simulink model "o1_ar_filter"  (R2020b)
settings: Solver=FixedStepDiscrete  StartTime=0.0  StopTime=stopTime  RelTol=1e-3
undefined symbols (not defined in the file or in its folder): fs
settings Model: Creator=Ross  LastModifiedBy=conno
settings DataIOCC: SaveOutput=off  SaveTime=off  ReturnWorkspaceOutputs=off
settings OptimizationCC: BlockReduction=off  ConditionallyExecuteInputs=off  DefaultParameterBehavior=Inlined
settings DebuggingCC: ReadBeforeWriteMsg=DisableAll  WriteAfterWriteMsg=DisableAll  WriteAfterReadMsg=DisableAll  AlgebraicLoopMsg=error  MultiTaskDSMMsg=none  SingleTaskRateTransMsg=error  PregeneratedLibrarySubsystemCodeDiagnostic=none  ArithmeticOperatorsInVariantConditions=warning
settings HardwareCC: ProdBitPerPointer=32  ProdBitPerSizeT=32  ProdBitPerPtrDiffT=32  ProdLargestAtomicFloat=None  ProdIntDivRoundTo=Undefined  ProdEndianess=Unspecified  ProdWordSize=32  ProdHWDeviceType=ASIC/FPGA->ASIC/FPGA  TargetBitPerPointer=64  TargetBitPerSizeT=64  TargetBitPerPtrDiffT=64  TargetLongLongMode=on  TargetIntDivRoundTo=Zero  TargetEndianess=LittleEndian  TargetWordSize=64  TargetHWDeviceType=Custom Processor->MATLAB Host Computer  ProdEqTarget=off
settings ModelReferenceCC: UpdateModelReferenceTargets=IfOutOfDate
settings SFSimCC: SFSimEcho=off  SimUseLocalCustomCode=off  CustomCodeUndefinedFunction=UseInterfaceOnly
settings RTWCC: RTWUseLocalCustomCode=off

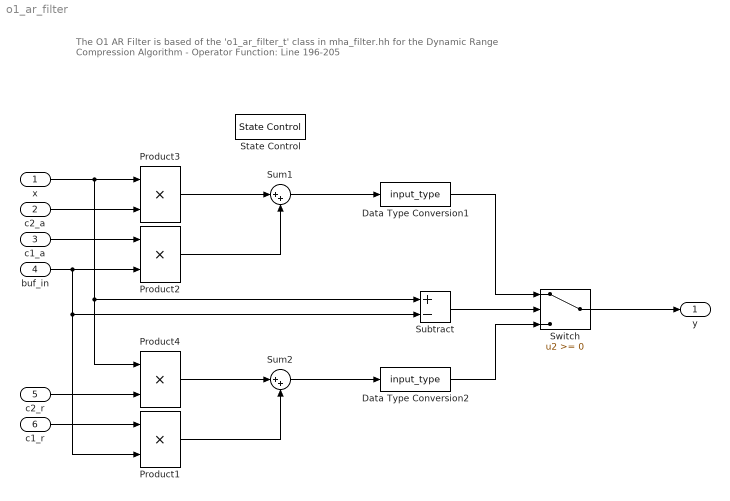
== system o1_ar_filter ==
  note: The O1 AR Filter is based of the 'o1_ar_filter_t' class in mha_filter.hh for the Dynamic Range Compression Algorithm
      | - Operator Function: Line 196-205
  x : Inport  OutDataTypeStr=input_type  SampleTime=1/fs
  c2_a : Inport  Port=2  OutDataTypeStr=ad_coeff_type
  c1_a : Inport  Port=3  OutDataTypeStr=ad_coeff_type
  buf_in : Inport  Port=4  OutDataTypeStr=input_type
  c2_r : Inport  Port=5  OutDataTypeStr=ad_coeff_type
  c1_r : Inport  Port=6  OutDataTypeStr=ad_coeff_type
  Data Type Conversion1 : DataTypeConversion  OutDataTypeStr=input_type  RndMeth=Nearest
  Data Type Conversion2 : DataTypeConversion  OutDataTypeStr=input_type  RndMeth=Nearest
  Product{1..4} (4 alike) : Product
  State Control : StateControl  StateControl=Synchronous
  Subtract : Sum  Inputs=+-
  Sum1 : Sum  Inputs=|++  OutDataTypeStr=Inherit: Same as first input
  Sum2 : Sum  Inputs=|++  OutDataTypeStr=Inherit: Same as first input
  Switch : Switch
  y : Outport
  wires:
  Product3/1 -> Sum1/1
  Product2/1 -> Sum1/2
  c2_a/1 -> Product3/2
  buf_in/1 -> Subtract/2, Product1/2, Product2/2
  c1_a/1 -> Product2/1
  x/1 -> Subtract/1, Product4/1, Product3/1
  Sum1/1 -> Data Type Conversion1/1
  c1_r/1 -> Product1/1
  c2_r/1 -> Product4/2
  Sum2/1 -> Data Type Conversion2/1
  Product4/1 -> Sum2/1
  Product1/1 -> Sum2/2
  Subtract/1 -> Switch/2
  Data Type Conversion2/1 -> Switch/3
  Data Type Conversion1/1 -> Switch/1
  Switch/1 -> y/1
